simulink model "FG_RealTime"  (R2017b)
settings: Solver=FixedStepDiscrete  StartTime=0.0  StopTime=inf  FixedStep=0.0005  RelTol=1e-3  EnableMultiTasking=on
InitFcn:
  | isSim = 0;
  | PreFunctions.CustomInitFcn;
libraries: slrtlib x2, CassieLibrary x1, Cassie_CommandBlock_Library_5 x1
settings Model: xpc_rtwmakecfg_data=_xpcethercatlib_  TunableVars=c_CovPos_abduction,c_CovPos_knee,c_CovPos_qj1,c_CovPos_qj2,c_CovPos_qj3,c_CovPos_rotation,c_CovPos_thigh,c_CovPos_toe,c_CovVel_abduction,c_CovVel_knee,c_CovVel_qj1,c_CovVel_qj2,c_CovVel_qj3,c_CovVel_rotation,c_CovVel_thigh,c_CovVel_toe,c_Cov_AngularVelocity,c_Cov_Euler,c_Cov_Euler_rates,c_Cov_LinearAccelerator_xy,c_Cov_LinearAccelerator_z,c_Cov_Lx_LRToe_stTD0,c_Cov_Ly_LRToe_stTD0,c_Cov_Orientation,c_Cov_rpx_LRToe_body,c_Cov_rpx_LRToe_stTD0,c_Cov_rpy_LRToe_body,c_Cov_rpy_LRToe_stTD0,c_Cov_rpz_LRToe_body,c_H_fil_param,c_IK_max_iter_num,c_Kd_abduction,c_Kd_knee,c_Kd_pitch,c_Kd_roll,c_Kd_rotation,c_Kd_st_rotation,c_Kd_thigh,c_Kd_toe,c_Kd_yaw,c_Kp_abduction,c_Kp_knee,c_Kp_pitch,c_Kp_roll,c_Kp_rotation,c_Kp_st_rotation,c_Kp_thigh,c_Kp_toe,c_Kp_yaw,c_KsL_1,c_KsL_2,c_KsR_1,c_KsR_2,c_Tx_slide_toe_2,c_Ty_slide_toe_2,c_Tz_slide_toe_2,c_Vx_tgd_fil_param,c_Vx_tgd_offset,c_Vy_tgd_avg_fil_param,c_Vy_tgd_offset,c_adjusted_desired_roll_angle_fil_param,c_com_x_offset,c_desired_com2stToe_lateral_fil_param,c_dop,c_history_length,c_knee_cp_time,c_lateral_correction_gain,c_max_st_rotation_motor_torque,c_max_turn_per_sec,c_one_step_max_vel_gain,c_rp_LRToe_fil_param,c_st_rotation_torque_ramp_time,c_stance_thre_lb,c_stance_thre_lb_2,c_stance_thre_ub,c_stance_thre_ub_2,c_toe_leave_ground_lb,c_toe_leave_ground_ub,c_torque_transition_time,c_u_abduction_swing_cp,c_u_knee_cp,c_u_pitch_cp,c_u_roll_cp,c_use_dq_AR_for_PD,c_vx_slide_toe_1,c_vx_slide_toe_2,c_vy_slide_toe_1,c_vy_slide_toe_2,c_vz_slide_toe_1,c_vz_slide_toe_2,c_yaw_error_fil_param  TunableVarsStorageClass=Auto,Auto,Auto,Auto,Auto,Auto,Auto,Auto,Auto,Auto,Auto,Auto,Auto,Auto,Auto,Auto,Auto,Auto,Auto,Auto,Auto,Auto,Auto,Auto,Auto,Auto,Auto,Auto,Auto,Auto,Auto,Auto,Auto,Auto,Auto,Auto,Auto,Auto,Auto,Auto,Auto,Auto,Auto,Auto,Auto,Auto,Auto,Auto,Auto,Auto,Auto,Auto,Auto,Auto,Auto,Auto,Auto,Auto,Auto,Auto,Auto,Auto,Auto,Auto,Auto,Auto,Auto,Auto,Auto,Auto,Auto,Auto,Auto,Auto,Auto,Auto,Auto,Auto,Auto,Auto,Auto,Auto,Auto,Auto,Auto,Auto,Auto,Auto,Auto,Auto,Auto  TunableVarsTypeQualifier=,,,,,,,,,,,,,,,,,,,,,,,,,,,,,,,,,,,,,,,,,,,,,,,,,,,,,,,,,,,,,,,,,,,,,,,,,,,,,,,,,,,,,,,,,,  Creator=robot  LastModifiedBy=81068
settings DataIOCC: SaveFormat=Array  SaveOutput=off  SignalLogging=off  DSMLogging=off  VisualizeSimOutput=off  SaveTime=off
settings OptimizationCC: LifeSpan=inf  SimCompilerOptimization=on  AccelVerboseBuild=on
settings DebuggingCC: AllowSymbolicDim=off  SFUnexpectedBacktrackingDiag=warning  SFNoUnconditionalDefaultTransitionDiag=warning  SFExecutionAtInitializationDiag=none
settings HardwareCC: ProdBitPerPointer=32  ProdBitPerSizeT=32  ProdBitPerPtrDiffT=32  ProdLargestAtomicFloat=None  ProdWordSize=32  ProdLongLongMode=on  ProdHWDeviceType=Generic->32-bit x86 compatible
settings ModelReferenceCC: ParallelModelReferenceMATLABWorkerInit=Copy Base Workspace  ModelReferenceNumInstancesAllowed=Zero  PropagateSignalLabelsOutOfModel=off
settings SFSimCC: SimUserIncludeDirs=$root_dir$\CustomCodes\utils\funcs\KinDyn200511_221619  SFSimEcho=off
settings SFSimCC: SimUserSources=|
  | R_LeftAbductionJoint_src.c
  | R_LeftThighJoint_src.c
  | R_RightAbductionJoint_src.c
  | R_RightThighJoint_src.c
  | 
  | AMworld_about_pA_src.c
  | 
  | Jb_BasePosX_src.c
  | Jb_BasePosY_src.c
  | Jb_BasePosZ_src.c
  | Jb_BaseRotX_src.c
  | Jb_BaseRotY_src.c
  | Jb_BaseRotZ_src.c
  | Jb_LeftAbductionJoint_src.c
  | Jb_LeftAnkleJoint_src.c
  | Jb_LeftHip_src.c
  | Jb_LeftKneeJoint_src.c
  | Jb_LeftKneeSpringJoint_src.c
  | Jb_LeftKnee_src.c
  | Jb_LeftPelvisRotation_src.c
  | Jb_LeftRotationJoint_src.c
  | Jb_LeftShin_src.c
  | Jb_LeftTarsus_src.c
  | Jb_LeftThighJoint_src.c
  | Jb_LeftThigh_src.c
  | Jb_LeftToeBottomBack_src.c
  | Jb_LeftToeBottomFront_src.c
  | Jb_LeftToeBottom_src.c
  | Jb_LeftToeJoint_src.c
  | Jb_LeftToe_src.c
  | Jb_Pelvis_src.c
  | Jb_RightAbductionJoint_src.c
  | Jb_RightAnkleJoint_src.c
  | Jb_RightHip_src.c
  | Jb_RightKneeJoint_src.c
  | Jb_RightKneeSpringJoint_src.c
  | Jb_RightKnee_src.c
  | Jb_RightPelvisRotation_src.c
  | Jb_RightRotationJoint_src.c
  | Jb_RightShin_src.c
  | Jb_RightTarsus_src.c
  | Jb_RightThighJoint_src.c
  | Jb_RightThigh_src.c
  | Jb_RightToeBottomBack_src.c
  | Jb_RightToeBottomFront_src.c
  | Jb_RightToeBottom_src.c
  | Jb_RightToeJoint_src.c
  | Jb_RightToe_src.c
  | 
  | Jdq_AMworld_about_pA_src.c
  | 
  | 
  | Jp_COM_src.c
  | Jp_LeftAbductionJoint_src.c
  | Jp_LeftAnkleJoint_src.c
  | Jp_LeftHip_src.c
  | Jp_LeftKneeJoint_src.c
  | Jp_LeftKneeSpringJoint_src.c
  | Jp_LeftKnee_src.c
  | Jp_LeftPelvisRotation_src.c
  | Jp_LeftRotationJoint_src.c
  | Jp_LeftShin_src.c
  | Jp_LeftTarsus_src.c
  | Jp_LeftThighJoint_src.c
  | Jp_LeftThigh_src.c
  | Jp_LeftToeBottomBack_src.c
  | Jp_LeftToeBottomFront_src.c
  | Jp_LeftToeBottom_src.c
  | Jp_LeftToeJoint_src.c
  | Jp_LeftToe_src.c
  | Jp_Pelvis_src.c
  | Jp_RightAbductionJoint_src.c
  | Jp_RightAnkleJoint_src.c
  | Jp_RightHip_src.c
  | Jp_RightKneeJoint_src.c
  | Jp_RightKneeSpringJoint_src.c
  | Jp_RightKnee_src.c
  | Jp_RightPelvisRotation_src.c
  | Jp_RightRotationJoint_src.c
  | Jp_RightShin_src.c
  | Jp_RightTarsus_src.c
  | Jp_RightThighJoint_src.c
  | Jp_RightThigh_src.c
  | Jp_RightToeBottomBack_src.c
  | Jp_RightToeBottomFront_src.c
  | Jp_RightToeBottom_src.c
  | Jp_RightToeJoint_src.c
  | Jp_RightToe_src.c
  | 
  | p_BasePosX_src.c
  | p_BasePosY_src.c
  | p_BasePosZ_src.c
  | p_BaseRotX_src.c
  | p_BaseRotY_src.c
  | p_BaseRotZ_src.c
  | p_COM_src.c
  | p_LeftAbductionJoint_src.c
  | p_LeftAnkleJoint_src.c
  | p_LeftHip_src.c
  | p_LeftKneeJoint_src.c
  | p_LeftKneeSpringJoint_src.c
  | p_LeftKnee_src.c
  | p_LeftPelvisRotation_src.c
  | p_LeftRotationJoint_src.c
  | p_LeftShin_src.c
  | p_LeftTarsus_src.c
  | p_LeftThighJoint_src.c
  | p_LeftThigh_src.c
  | p_LeftToeBottomBack_src.c
  | p_LeftToeBottomFront_src.c
  | p_LeftToeBottom_src.c
  | p_LeftToeJoint_src.c
  | p_LeftToe_src.c
  | p_Pelvis_src.c
  | p_RightAbductionJoint_src.c
  | p_RightAnkleJoint_src.c
  | p_RightHip_src.c
  | p_RightKneeJoint_src.c
  | p_RightKneeSpringJoint_src.c
  | p_RightKnee_src.c
  | p_RightPelvisRotation_src.c
  | p_RightRotationJoint_src.c
  | p_RightShin_src.c
  | p_RightTarsus_src.c
  | p_RightThighJoint_src.c
  | p_RightThigh_src.c
  | p_RightToeBottomBack_src.c
  | p_RightToeBottomFront_src.c
  | p_RightToeBottom_src.c
  | p_RightToeJoint_src.c
  | p_RightToe_src.c
  | 
  | T_LeftToeBottomBack_src.c
  | T_LeftToeBottomFront_src.c
  | T_LeftToeBottom_src.c
  | T_RightToeBottomBack_src.c
  | T_RightToeBottomFront_src.c
  | T_RightToeBottom_src.c
  | 
  | J_LL_Left_src.c
  | J_LL_Right_src.c
  | LL_Left_src.c
  | LL_Right_src.c
settings RTWCC: SystemTargetFile=slrt.tlc  TLCOptions=-axPCMaxOverloads=1000000000 -axPCMaxOverloadLen=1000000000  TemplateMakefile=slrt_default_tmf  Description=Simulink Real-Time  RTWUseSimCustomCode=on  CustomInclude=$root_dir$\CustomCodes\utils\funcs\KinDyn200511_221619  CodeExecutionProfiling=on  RTWCompilerOptimization=on
settings RTWCC: CustomSource=|
  | R_LeftAbductionJoint_src.c
  | R_LeftThighJoint_src.c
  | R_RightAbductionJoint_src.c
  | R_RightThighJoint_src.c
  | 
  | AMworld_about_pA_src.c
  | 
  | Jb_BasePosX_src.c
  | Jb_BasePosY_src.c
  | Jb_BasePosZ_src.c
  | Jb_BaseRotX_src.c
  | Jb_BaseRotY_src.c
  | Jb_BaseRotZ_src.c
  | Jb_LeftAbductionJoint_src.c
  | Jb_LeftAnkleJoint_src.c
  | Jb_LeftHip_src.c
  | Jb_LeftKneeJoint_src.c
  | Jb_LeftKneeSpringJoint_src.c
  | Jb_LeftKnee_src.c
  | Jb_LeftPelvisRotation_src.c
  | Jb_LeftRotationJoint_src.c
  | Jb_LeftShin_src.c
  | Jb_LeftTarsus_src.c
  | Jb_LeftThighJoint_src.c
  | Jb_LeftThigh_src.c
  | Jb_LeftToeBottomBack_src.c
  | Jb_LeftToeBottomFront_src.c
  | Jb_LeftToeBottom_src.c
  | Jb_LeftToeJoint_src.c
  | Jb_LeftToe_src.c
  | Jb_Pelvis_src.c
  | Jb_RightAbductionJoint_src.c
  | Jb_RightAnkleJoint_src.c
  | Jb_RightHip_src.c
  | Jb_RightKneeJoint_src.c
  | Jb_RightKneeSpringJoint_src.c
  | Jb_RightKnee_src.c
  | Jb_RightPelvisRotation_src.c
  | Jb_RightRotationJoint_src.c
  | Jb_RightShin_src.c
  | Jb_RightTarsus_src.c
  | Jb_RightThighJoint_src.c
  | Jb_RightThigh_src.c
  | Jb_RightToeBottomBack_src.c
  | Jb_RightToeBottomFront_src.c
  | Jb_RightToeBottom_src.c
  | Jb_RightToeJoint_src.c
  | Jb_RightToe_src.c
  | 
  | Jdq_AMworld_about_pA_src.c
  | 
  | 
  | Jp_COM_src.c
  | Jp_LeftAbductionJoint_src.c
  | Jp_LeftAnkleJoint_src.c
  | Jp_LeftHip_src.c
  | Jp_LeftKneeJoint_src.c
  | Jp_LeftKneeSpringJoint_src.c
  | Jp_LeftKnee_src.c
  | Jp_LeftPelvisRotation_src.c
  | Jp_LeftRotationJoint_src.c
  | Jp_LeftShin_src.c
  | Jp_LeftTarsus_src.c
  | Jp_LeftThighJoint_src.c
  | Jp_LeftThigh_src.c
  | Jp_LeftToeBottomBack_src.c
  | Jp_LeftToeBottomFront_src.c
  | Jp_LeftToeBottom_src.c
  | Jp_LeftToeJoint_src.c
  | Jp_LeftToe_src.c
  | Jp_Pelvis_src.c
  | Jp_RightAbductionJoint_src.c
  | Jp_RightAnkleJoint_src.c
  | Jp_RightHip_src.c
  | Jp_RightKneeJoint_src.c
  | Jp_RightKneeSpringJoint_src.c
  | Jp_RightKnee_src.c
  | Jp_RightPelvisRotation_src.c
  | Jp_RightRotationJoint_src.c
  | Jp_RightShin_src.c
  | Jp_RightTarsus_src.c
  | Jp_RightThighJoint_src.c
  | Jp_RightThigh_src.c
  | Jp_RightToeBottomBack_src.c
  | Jp_RightToeBottomFront_src.c
  | Jp_RightToeBottom_src.c
  | Jp_RightToeJoint_src.c
  | Jp_RightToe_src.c
  | 
  | p_BasePosX_src.c
  | p_BasePosY_src.c
  | p_BasePosZ_src.c
  | p_BaseRotX_src.c
  | p_BaseRotY_src.c
  | p_BaseRotZ_src.c
  | p_COM_src.c
  | p_LeftAbductionJoint_src.c
  | p_LeftAnkleJoint_src.c
  | p_LeftHip_src.c
  | p_LeftKneeJoint_src.c
  | p_LeftKneeSpringJoint_src.c
  | p_LeftKnee_src.c
  | p_LeftPelvisRotation_src.c
  | p_LeftRotationJoint_src.c
  | p_LeftShin_src.c
  | p_LeftTarsus_src.c
  | p_LeftThighJoint_src.c
  | p_LeftThigh_src.c
  | p_LeftToeBottomBack_src.c
  | p_LeftToeBottomFront_src.c
  | p_LeftToeBottom_src.c
  | p_LeftToeJoint_src.c
  | p_LeftToe_src.c
  | p_Pelvis_src.c
  | p_RightAbductionJoint_src.c
  | p_RightAnkleJoint_src.c
  | p_RightHip_src.c
  | p_RightKneeJoint_src.c
  | p_RightKneeSpringJoint_src.c
  | p_RightKnee_src.c
  | p_RightPelvisRotation_src.c
  | p_RightRotationJoint_src.c
  | p_RightShin_src.c
  | p_RightTarsus_src.c
  | p_RightThighJoint_src.c
  | p_RightThigh_src.c
  | p_RightToeBottomBack_src.c
  | p_RightToeBottomFront_src.c
  | p_RightToeBottom_src.c
  | p_RightToeJoint_src.c
  | p_RightToe_src.c
  | 
  | T_LeftToeBottomBack_src.c
  | T_LeftToeBottomFront_src.c
  | T_LeftToeBottom_src.c
  | T_RightToeBottomBack_src.c
  | T_RightToeBottomFront_src.c
  | T_RightToeBottom_src.c
  | 
  | J_LL_Left_src.c
  | J_LL_Right_src.c
  | LL_Left_src.c
  | LL_Right_src.c
settings CodeAppCC: GenerateComments=off  MaxIdLength=128  SimulinkBlockComments=off
settings ConfigComp: CovMetricSettings=dw  CovHtmlReporting=on  CovSaveCumulativeToWorkspaceVar=on  CovSaveSingleToWorkspaceVar=on  CovExternalEMLEnable=off

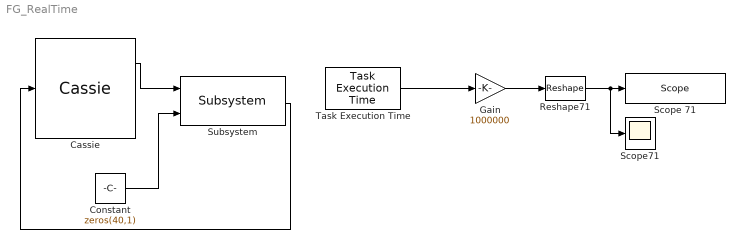
== system FG_RealTime ==
  Cassie : CassieLibrary/RealTime/Cassie  SystemSampleTime=-1
  Constant : Constant  Value=zeros(40,1)
  Gain : Gain  Gain=1000000
  Reshape71 : Reshape
  Scope 71 : slrtlib/Displays and Logging/Scope   scopeno=1234  scopetype=Host  autostart=on  viewmode=Graphical redraw  formatstr='%15.6f'  grid=on  ylimits=[0,0]  nosamples=2500  noprepostsamples=0  interleave=1  triggermode=FreeRun  triggersignal=1  trigsignalfromport=off  triggerlevel=0.0  triggerslope=Either  triggerscope=1  triggersample=0  filename=data.dat  mode=Lazy  writesize=512  autorestart=off  dynamicfilemode=off  maxwritefilesize=512*1024^2
  Scope71 : Scope
  Subsystem : Cassie_CommandBlock_Library_5/Subsystem
  "Task Execution Time " : slrtlib/Target Management/Execution Parameters/Task Execution Time   ts=0.0005
      settings: SourceProductName=Simulink Real-Time  SourceProductBaseCode=XP
  wires:
  Subsystem/1 -> Cassie/1
  Cassie/1 -> Subsystem/1
  Reshape71/1 -> Scope71/1, Scope 71/1
  "Task Execution Time "/1 -> Gain/1
  Gain/1 -> Reshape71/1
  Constant/1 -> Subsystem/2
